simulink model "Heli_outer_loop"  (R2019a)
settings: Solver=FixedStepDiscrete  StartTime=0.0  StopTime=10.0  FixedStep=0.01  RelTol=1e-3  EnableMultiTasking=on
undefined symbols (not defined in the file or in its folder): DiscIntNeverNeededParam
libraries: simulink x1
Description:
  | This model implements the outer loop control for a helicopter.  Based on pilot inputs the outer loop control pitch attitude, roll attitude and yaw rate.
settings Model: DataDictionary=HeliSystemDD.sldd  Creator=bpotter  LastModifiedBy=bpotter
settings DataIOCC: LimitDataPoints=on  SaveFormat=Array
settings OptimizationCC: BlockReduction=off  DefaultParameterBehavior=Inlined  UseDivisionForNetSlopeComputation=on  InitFltsAndDblsToZero=on  EfficientFloat2IntCast=on  EfficientMapNaN2IntZero=off  LifeSpan=inf  MaxStackSize=inf
settings DebuggingCC: SignalInfNanChecking=error  SignalRangeChecking=error  ReadBeforeWriteMsg=EnableAllAsError  WriteAfterWriteMsg=EnableAllAsError  WriteAfterReadMsg=EnableAllAsError  AlgebraicLoopMsg=error  ArtificialAlgebraicLoopMsg=error  SaveWithDisabledLinksMsg=error  SaveWithParameterizedLinksMsg=error  BlockPriorityViolationMsg=error  SolverPrmCheckMsg=error  InheritedTsInSrcMsg=error  SingleTaskRateTransMsg=error  TasksWithSamePriorityMsg=error  SigSpecEnsureSampleTimeMsg=error  CheckMatrixSingularityMsg=error  IntegerOverflowMsg=error  ParameterUnderflowMsg=error  ParameterPrecisionLossMsg=error  ParameterTunabilityLossMsg=error  UnderSpecifiedDataTypeMsg=error  UnnecessaryDatatypeConvMsg=warning  VectorMatrixConversionMsg=error  SignalLabelMismatchMsg=error  UnconnectedInputMsg=error  UnconnectedOutputMsg=error  UnconnectedLineMsg=error  SFcnCompatibilityMsg=error  UniqueDataStoreMsg=error  BusObjectLabelMismatch=error  RootOutportRequireBusObject=error  AssertControl=DisableAll  AllowSymbolicDim=off  ModelReferenceIOMsg=error  ModelReferenceIOMismatchMessage=error  UnknownTsInhSupMsg=error  ModelReferenceDataLoggingMessage=error  StateNameClashWarn=warning  PregeneratedLibrarySubsystemCodeDiagnostic=none  StrictBusMsg=ErrorOnBusTreatedAsVector  NonBusSignalsTreatedAsBus=error  SFInvalidInputDataAccessInChartInitDiag=error  SFTransitionOutsideNaturalParentDiag=error  SFUnreachableExecutionPathDiag=error  SFUndirectedBroadcastEventsDiag=error  SFTransitionActionBeforeConditionDiag=error  SFExecutionAtInitializationDiag=none  IntegerSaturationMsg=error  ArithmeticOperatorsInVariantConditions=warning
settings HardwareCC: ProdBitPerPointer=32  ProdBitPerSizeT=32  ProdBitPerPtrDiffT=32  ProdWordSize=32  ProdHWDeviceType=Intel->x86-32 (Windows32)  TargetIntDivRoundTo=Zero
settings ModelReferenceCC: ModelReferenceNumInstancesAllowed=Single  PropagateSignalLabelsOutOfModel=off
settings SFSimCC: SimUseLocalCustomCode=off  CompileTimeRecursionLimit=0  EnableRuntimeRecursion=off  MATLABDynamicMemAlloc=off
settings RTWCC: SystemTargetFile=ert.tlc  TemplateMakefile=ert_default_tmf  GenerateReport=on  RTWUseLocalCustomCode=off  IncludeHyperlinkInReport=on  LaunchReport=on  PortableWordSizes=on  GenerateTraceInfo=on  GenerateTraceReport=on  GenerateTraceReportSl=on  GenerateTraceReportSf=on  GenerateTraceReportEml=on
settings CodeAppCC: ForceParamTrailComments=on  IgnoreCustomStorageClasses=off  MATLABFcnDesc=on  MangleLength=4  StateflowObjectComments=on  ReqsInCode=on
settings ERTTargetCC: TargetLangStandard=C99 (ISO)  UtilityFuncGeneration=Shared location  MultiwordLength=2048  GenerateSampleERTMain=on  IncludeMdlTerminateFcn=off  SuppressErrorStatus=on  SupportAbsoluteTime=off  SupportNonFinite=off  ParenthesesLevel=Maximum  CastingMode=Standards  GenerateSharedConstants=off  ERTCustomFileTemplate=example_file_process.tlc  ERTFilePackagingFormat=Compact  PreserveExpressionOrder=on  PreserveIfCondition=on  ConvertIfToSwitch=off  SuppressUnreachableDefaultCases=off  EnableSignedLeftShifts=off  EnableSignedRightShifts=off
settings ConfigComp: CovMetricSettings=dw  CovHtmlReporting=on  CovSaveCumulativeToWorkspaceVar=on  CovSaveSingleToWorkspaceVar=on  CovExternalEMLEnable=off  CovSFcnEnable=off  PSVerificationMode=BugFinder  PSResultDir=BugFinder_results_$ModelName$  PSAutoStubLUT=off

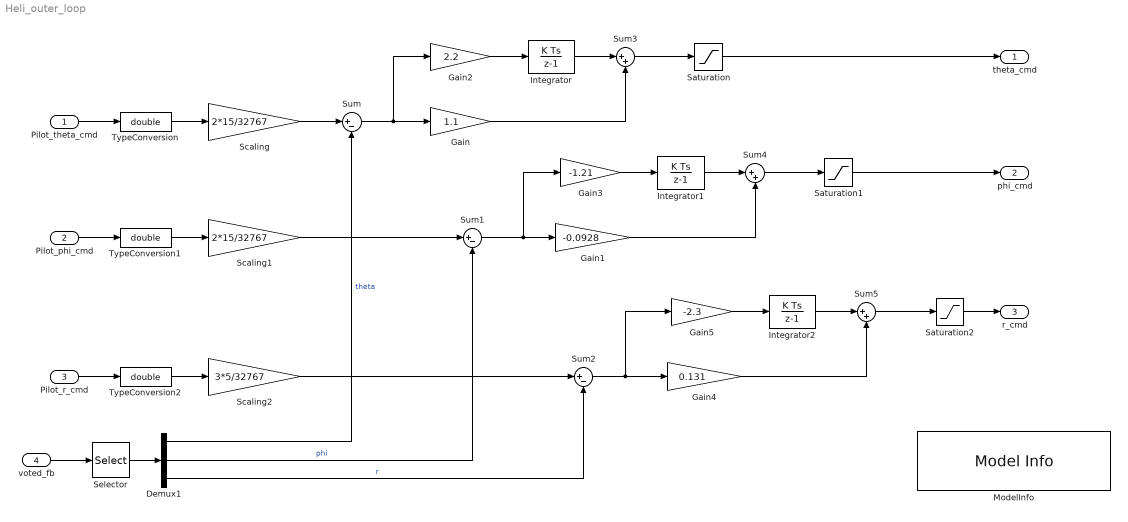
== system Heli_outer_loop ==
  Pilot_theta_cmd : Inport  RequirementInfo={} %GIDa_c6e8f1b9_b611_43b0_b09b_f7299b128b80  OutMin=-32768  OutMax=32767  OutDataTypeStr=int16  PortDimensions=1  SampleTime=0.01
  Pilot_phi_cmd : Inport  RequirementInfo={} %GIDa_de5a2227_6f1d_448c_bc8c_e667ffb26dd8  Port=2  OutMin=-32768  OutMax=32767  OutDataTypeStr=int16  PortDimensions=1  SampleTime=0.01
  Pilot_r_cmd : Inport  RequirementInfo={} %GIDa_bd336e52_072b_4081_8e24_5224b916f056  Port=3  OutMin=-32768  OutMax=32767  OutDataTypeStr=int16  PortDimensions=1  SampleTime=0.01
  voted_fb : Inport  RequirementInfo={} %GIDa_40b9d006_7ccb_49cb_a6ac_aff381845bc4  Port=4  OutMin=-180  OutMax=180  OutDataTypeStr=double  PortDimensions=5  SampleTime=0.01
  Demux1 : Demux  RequirementInfo={} %GIDa_0f7e0ef4_98d4_4326_93b8_613d0164b4b2  Outputs=3
  Gain : Gain  RequirementInfo={} %GIDa_38b33631_7d46_423a_acdb_ff93985993a9  Gain=1.1
  Gain1 : Gain  RequirementInfo={} %GIDa_225d17d5_1a8e_4842_95f8_ce528d38517d  Gain=-0.0928
  Gain2 : Gain  RequirementInfo={} %GIDa_ec453ec5_c5c0_44d5_948e_65c93ddaef7c  Gain=2.2
  Gain3 : Gain  RequirementInfo={} %GIDa_943f3cbe_3937_44aa_af38_ec7fec40805c  Gain=-1.21
  Gain4 : Gain  RequirementInfo={} %GIDa_d845b47e_971b_498b_bbe3_d6058df44643  Gain=0.131
  Gain5 : Gain  RequirementInfo={} %GIDa_0a451155_7422_4e41_b41b_ac8de7a0f7bc  Gain=-2.3
  Integrator : DiscreteIntegrator  RequirementInfo={} %GIDa_dac8ce2c_b2e5_46af_8a5f_5c149ac95a38  SampleTime=-1  LimitOutput=on  UpperSaturationLimit=10  LowerSaturationLimit=-10  ICPrevOutput=DiscIntNeverNeededParam  ICPrevScaledInput=DiscIntNeverNeededParam
      settings: AttributesFormatString="%<LowerSaturationLimit> to  %<UpperSaturationLimit>"
  Integrator1 : DiscreteIntegrator  RequirementInfo={} %GIDa_c2996118_add0_406e_b8f4_096077f2e691  SampleTime=-1  LimitOutput=on  UpperSaturationLimit=10  LowerSaturationLimit=-10  ICPrevOutput=DiscIntNeverNeededParam  ICPrevScaledInput=DiscIntNeverNeededParam
      settings: AttributesFormatString="%<LowerSaturationLimit> to  %<UpperSaturationLimit>"
  Integrator2 : DiscreteIntegrator  RequirementInfo={} %GIDa_cf0bee46_0c0a_47b2_81ab_c926ffb37de9  SampleTime=-1  LimitOutput=on  UpperSaturationLimit=10  LowerSaturationLimit=-10  ICPrevOutput=DiscIntNeverNeededParam  ICPrevScaledInput=DiscIntNeverNeededParam
      settings: AttributesFormatString="%<LowerSaturationLimit> to  %<UpperSaturationLimit>"
  ModelInfo : simulink/Model-Wide Utilities/Model Info  Frame=on  DisplayStringWithTags=|  HorizontalTextAlignment=Center  LeftAlignmentValue=0.5
      | Model Name: %<ModelName>
      | Model Version: %<ModelVersion>
      | Last Modified: %<LastModificationDate>
      | 
      | Copyright 2016 The MathWorks, Inc.
  Saturation : Saturate  RequirementInfo={} %GIDa_cd349ed3_fa5b_45c3_8aec_effea4668e69  UpperLimit=30  LowerLimit=-30
      settings: AttributesFormatString=%<LowerLimit> to %<UpperLimit>
  Saturation1 : Saturate  RequirementInfo={} %GIDa_cdaf265c_9ec2_4b78_ae7f_0c72f3978ef0  UpperLimit=30  LowerLimit=-30
      settings: AttributesFormatString=%<LowerLimit> to %<UpperLimit>
  Saturation2 : Saturate  RequirementInfo={} %GIDa_b0697b07_104a_4fe5_acf7_d696411481f0  UpperLimit=30  LowerLimit=-30
      settings: AttributesFormatString=%<LowerLimit> to %<UpperLimit>
  Scaling : Gain  Gain=2*15/32767
  Scaling1 : Gain  Gain=2*15/32767
  Scaling2 : Gain  Gain=3*5/32767
  Selector : Selector  RequirementInfo={} %GIDa_e0faeade_0420_4977_bcc4_4057337ee888  InputPortWidth=5  IndexOptions=Index vector (dialog)  Indices=[1 2 3]  OutputSizes=1
  Sum : Sum  RequirementInfo={} %GIDa_aef1367a_fa96_4043_ad47_b91e9938bcbc  Inputs=|+-  InputSameDT=on  OutDataTypeStr=Inherit: Same as first input
  Sum1 : Sum  RequirementInfo={} %GIDa_7cf7cd4c_9daa_4c96_981c_13db01e8d568  Inputs=|+-  InputSameDT=on  OutDataTypeStr=Inherit: Same as first input
  Sum2 : Sum  RequirementInfo={} %GIDa_b75e5239_9c3e_4a2f_9dd4_07e5bc1f13e4  Inputs=|+-  InputSameDT=on  OutDataTypeStr=Inherit: Same as first input
  Sum3 : Sum  RequirementInfo={} %GIDa_dec0004f_1794_4f54_b78d_88f0915d9f6f  Inputs=|++
  Sum4 : Sum  RequirementInfo={} %GIDa_c73371f2_60d8_4f3a_a310_54a28eb8e7bc  Inputs=|++
  Sum5 : Sum  RequirementInfo={} %GIDa_e62dfe4c_4b0b_418d_84f2_d28db5a50898  Inputs=|++
  TypeConversion : DataTypeConversion  OutDataTypeStr=double
  TypeConversion1 : DataTypeConversion  OutDataTypeStr=double
  TypeConversion2 : DataTypeConversion  OutDataTypeStr=double
  theta_cmd : Outport  RequirementInfo={} %GIDa_56ddc0ff_d81c_44a6_a61d_90e8f701c995
  phi_cmd : Outport  RequirementInfo={} %GIDa_10908ca3_1080_4a03_a980_f863f0f9143a  Port=2
  r_cmd : Outport  RequirementInfo={} %GIDa_d0f1d3df_6d10_4b46_9cf8_3e0612fe178e  Port=3
  wires:
  Selector/1 -> Demux1/1
  Demux1/1 -> Sum/2  "theta"
  Demux1/2 -> Sum1/2  "phi"
  Demux1/3 -> Sum2/2  "r"
  voted_fb/1 -> Selector/1
  Sum/1 -> Gain/1, Gain2/1
  Gain/1 -> Sum3/2
  Sum3/1 -> Saturation/1
  Integrator/1 -> Sum3/1
  Gain2/1 -> Integrator/1
  Saturation/1 -> theta_cmd/1
  Sum1/1 -> Gain3/1, Gain1/1
  Gain1/1 -> Sum4/2
  Sum4/1 -> Saturation1/1
  Integrator1/1 -> Sum4/1
  Gain3/1 -> Integrator1/1
  Saturation1/1 -> phi_cmd/1
  Gain4/1 -> Sum5/2
  Sum5/1 -> Saturation2/1
  Integrator2/1 -> Sum5/1
  Gain5/1 -> Integrator2/1
  Sum2/1 -> Gain5/1, Gain4/1
  Saturation2/1 -> r_cmd/1
  TypeConversion2/1 -> Scaling2/1
  TypeConversion1/1 -> Scaling1/1
  TypeConversion/1 -> Scaling/1
  Pilot_theta_cmd/1 -> TypeConversion/1
  Scaling/1 -> Sum/1
  Pilot_phi_cmd/1 -> TypeConversion1/1
  Scaling1/1 -> Sum1/1
  Pilot_r_cmd/1 -> TypeConversion2/1
  Scaling2/1 -> Sum2/1
